simulink model "HW_2_FSR_EX4"  (R2023b)
settings: Solver=VariableStepAuto  StartTime=0.0  StopTime=tf  RelTol=1e-3
libraries: robotmobilelib x1
settings Model: Creator=Tony  LastModifiedBy=Tony
settings ModelReferenceCC: EnableRefExpFcnMdlSchedulingChecks=on

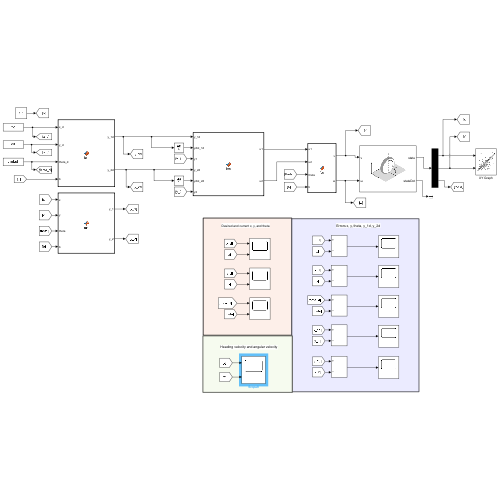
[thumbnail: Simulink's stored preview of the top-level diagram]
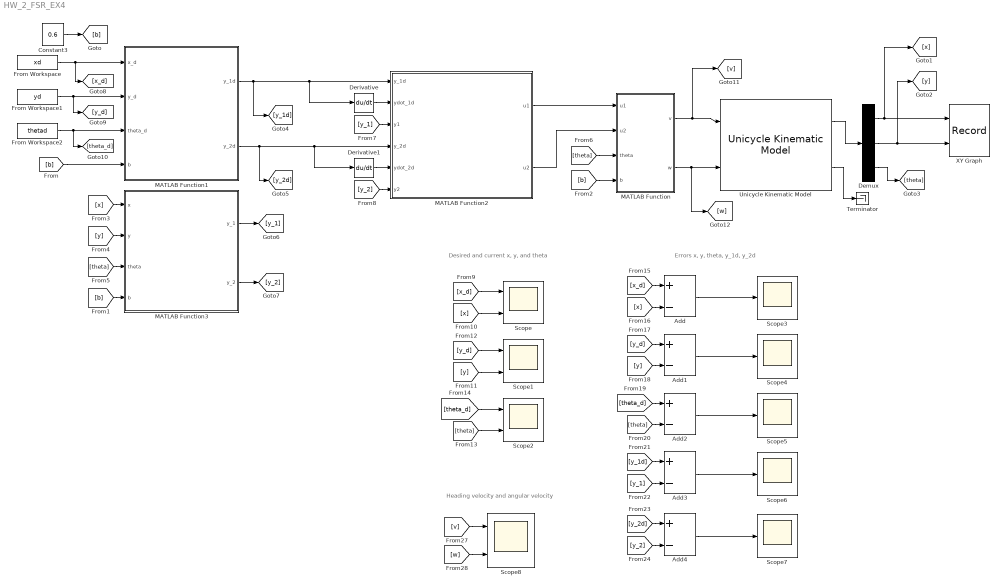
== system HW_2_FSR_EX4 ==
  note: Errors x, y, theta, y_1d, y_2d
  note: Desired and current x, y, and theta
  note: Heading velocity and angular velocity
  Add{,1..4} (5 alike) : Sum  Inputs=+-
  Constant3 : Constant  Value=0.6
  Demux : Demux  Outputs=3
  Derivative : Derivative
  Derivative1 : Derivative
  From Workspace : FromWorkspace  VariableName=xd
  From Workspace1 : FromWorkspace  VariableName=yd
  From Workspace2 : FromWorkspace  VariableName=thetad
  MATLAB Function : MATLAB Function  TreatAsAtomicUnit=on
  MATLAB Function1 : MATLAB Function  TreatAsAtomicUnit=on
  MATLAB Function2 : MATLAB Function  TreatAsAtomicUnit=on
  MATLAB Function3 : MATLAB Function  TreatAsAtomicUnit=on
  Scope{,1..2,8} (4 alike) : Scope  NumInputPorts=2
  Scope{3..7} (5 alike) : Scope
  Terminator : Terminator
  Unicycle Kinematic Model : robotmobilelib/Unicycle Kinematic Model  VehicleInputs=Vehicle Speed & Heading Angular Velocity  WheelRadius=0.1  WheelSpeedRange=[-Inf Inf]  InitialState=[0; 0; 0]  SimulateUsing=Interpreted execution
  XY Graph : Record  FileSettingsInternal="{\"entries\":[{\"content\":{\"excelSettings\":{\"content\":{},\"type\":\"Streamout.ExcelSettings\"}},\"type\":\"Streamout.FileSettingStorage\",\"uuid\":\"\"}],\"packageUris\":[\"http:\\/\\/schema.mathworks.com\\/mf0\\/streamout_blocks\\/R2020a\"],\"version\":\"1.0\"}"  Layout=[1 1]  SignalsInternal="{\"entries\":[{\"content\":{\"signals\":[{\"content\":{\"blockPath\":[],\"dimensions\":[1],\"domain\":\"\",\"lineColor\":\"#a2142f\",\"plots\":[ 1 ],\"port\":1,\"sid\":[\"\"],\"signalID\":1,\"signalName\":\"Demux:1\"},\"type\":\"RecordBlkView.Signal\",\"uuid\":\"\"},{\"content\":{\"blockPath\":[],\"dimensions\":[1],\"domain\":\"\",\"lineColor\":\"#139fff\",\"plots\":[ 1 ],\"port\":2,\"sid\":[\"\"],\"signalID\":2,\"signalName\":\"Demux:2\"},\"type\":\"RecordBlkView.Signal\",\"uuid\":\"\"}]},\"type\":\"RecordBlkView.InputSignals\",\"uuid\":\"\"}],\"packageUris\":[\"http:\\/\\/schema.mathworks.com\\/mf0\\/streamout_blocks\\/R2020a\"],\"version\":\"1.0\"}"  VisualizationBindings="{\"xyplotplugin\":{\"info\":[{\"series\":[{\"bindingParametersList\":[{\"parameter\":\"X-Axis\",\"signalID\":1,\"signalName\":\"Demux:1\"},{\"parameter\":\"Y-Axis\",\"signalID\":2,\"signalName\":\"Demux:2\"}],\"seriesID\":0}],\"subplotID\":1}]}}"  CompatibilityTag=XY
  wires:
  MATLAB Function/2(w) -> [w], Unicycle Kinematic Model/2
  From Workspace/1 -> [x_d], MATLAB Function1/1(x_d)
  From Workspace1/1 -> [y_d], MATLAB Function1/2(y_d)
  From Workspace2/1 -> [theta_d], MATLAB Function1/3(theta_d)
  Constant3/1 -> [b]
  [b] -> MATLAB Function1/4(b)
  MATLAB Function1/1(y_1d) -> [y_1d], Derivative/1, MATLAB Function2/1(y_1d)
  Derivative/1 -> MATLAB Function2/2(ydot_1d)
  Derivative1/1 -> MATLAB Function2/5(ydot_2d)
  MATLAB Function2/1(u1) -> MATLAB Function/1(u1)
  MATLAB Function2/2(u2) -> MATLAB Function/2(u2)
  Unicycle Kinematic Model/1 -> Demux/1
  [b] -> MATLAB Function3/4(b)
  [b] -> MATLAB Function/4(b)
  Demux/3 -> [theta]
  [x] -> MATLAB Function3/1(x)
  [y] -> MATLAB Function3/2(y)
  [theta] -> MATLAB Function3/3(theta)
  [theta] -> MATLAB Function/3(theta)
  MATLAB Function1/2(y_2d) -> [y_2d], Derivative1/1, MATLAB Function2/4(y_2d)
  MATLAB Function3/1(y_1) -> [y_1]
  MATLAB Function3/2(y_2) -> [y_2]
  [y_1] -> MATLAB Function2/3(y1)
  [y_2] -> MATLAB Function2/6(y2)
  [x_d] -> Scope/1
  [x] -> Scope/2
  [y_d] -> Scope1/1
  [y] -> Scope1/2
  [theta_d] -> Scope2/1
  [theta] -> Scope2/2
  [x_d] -> Add/1
  [x] -> Add/2
  Add/1 -> Scope3/1
  [y_d] -> Add1/1
  [y] -> Add1/2
  [theta_d] -> Add2/1
  [theta] -> Add2/2
  [y_1] -> Add3/2
  [y_1d] -> Add3/1
  [y_2] -> Add4/2
  [y_2d] -> Add4/1
  Demux/1 -> [x], XY Graph/1
  Demux/2 -> XY Graph/2, [y]
  MATLAB Function/1(v) -> [v], Unicycle Kinematic Model/1
  [v] -> Scope8/1
  [w] -> Scope8/2
  Unicycle Kinematic Model/2 -> Terminator/1
  Add1/1 -> Scope4/1
  Add2/1 -> Scope5/1
  Add3/1 -> Scope6/1
  Add4/1 -> Scope7/1

== matlab function HW_2_FSR_EX4/MATLAB Function1 ==
  data: x_d input; y_1d output; y_d input; theta_d input; y_2d output; b input
function [y_1d,y_2d]  = fcn(x_d,y_d,theta_d,b)

y_1d=x_d+b*cos(theta_d);
y_2d=y_d+b*sin(theta_d);

end

== matlab function HW_2_FSR_EX4/MATLAB Function ==
  data: u1 input; v output; w output; u2 input; theta input; b input
function [v,w] = fcn(u1,u2,theta,b)


T=[cos(theta) -b*sin(theta); sin(theta) b*cos(theta)];


Tinv = inv(T);

v = Tinv(1,:)*[u1; u2];
w = Tinv(2,:)*[u1; u2];

end

== matlab function HW_2_FSR_EX4/MATLAB Function2 ==
  data: y_1d input; u1 output; ydot_1d input; y1 input; y_2d input; ydot_2d input; y2 input; u2 output
function [u1,u2] = fcn(y_1d,ydot_1d,y1,y_2d,ydot_2d,y2)

k1=5;
k2=5;

u1=ydot_1d+k1*(y_1d-y1);
u2=ydot_2d+k2*(y_2d-y2);
end

== matlab function HW_2_FSR_EX4/MATLAB Function3 ==
  data: x input; y_1 output; y input; theta input; y_2 output; b input
function [y_1,y_2]  = fcn(x,y,theta,b)

y_1=x+b*cos(theta);
y_2=y+b*sin(theta);

end
